simulink model "exampleStorage_type4"  (R2016b)
settings: Solver=ode45  StartTime=0.0  StopTime=3*3600-2  RelTol=1e-3  EnableMultiTasking=on
libraries: carnot x14, simulink x4
settings Model: Creator=drhf  LastModifiedBy=drhf
settings DataIOCC: LimitDataPoints=on  SaveFormat=Array
settings OptimizationCC: ExpressionDepthLimit=2147483647  LifeSpan=inf
settings DebuggingCC: UnderspecifiedInitializationDetection=Classic  MergeDetectMultiDrivingBlocksExec=none  SolverPrmCheckMsg=warning  StateNameClashWarn=warning  SFUnexpectedBacktrackingDiag=warning  SFNoUnconditionalDefaultTransitionDiag=warning  SFExecutionAtInitializationDiag=none
settings HardwareCC: ProdBitPerPointer=32  ProdBitPerSizeT=32  ProdBitPerPtrDiffT=32  ProdLargestAtomicFloat=None  ProdIntDivRoundTo=Undefined  ProdEndianess=Unspecified  ProdWordSize=32  ProdHWDeviceType=32-bit Generic
settings ModelReferenceCC: PropagateSignalLabelsOutOfModel=off
settings GRTTargetCC: TargetLangStandard=C89/C90 (ANSI)  GeneratePreprocessorConditionals=Disable all  CombineOutputUpdateFcns=off  GRTInterface=on
settings ConfigComp: CovMetricSettings=dw  CovHtmlReporting=on  CovSaveCumulativeToWorkspaceVar=on  CovSaveSingleToWorkspaceVar=on  CovExternalEMLEnable=off

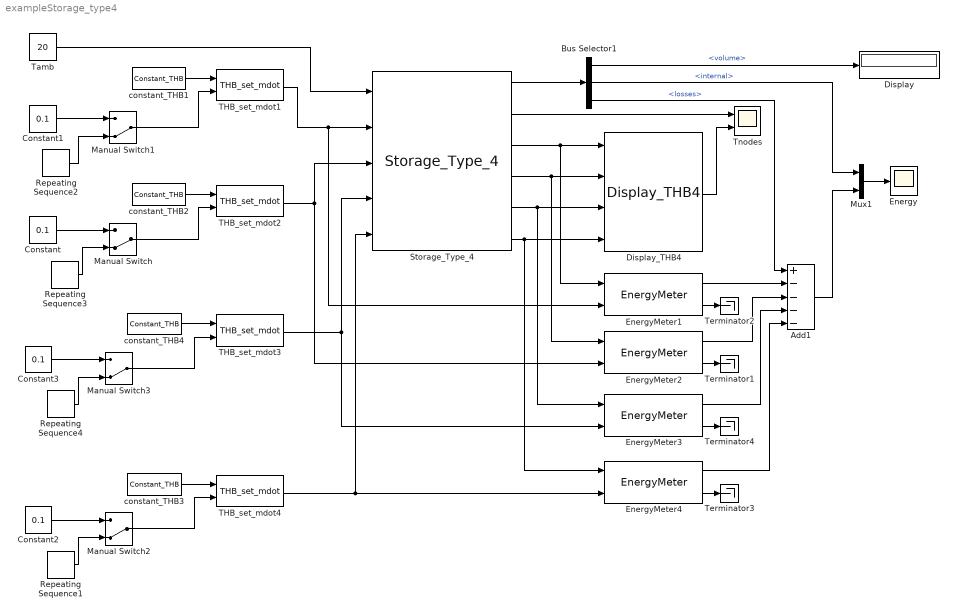
== system exampleStorage_type4 ==
  Add1 : Sum  Inputs=+----
  Bus Selector1 : BusSelector  OutputSignals=volume,energy.internal,energy.losses
  Constant{,1..3} (4 alike) : Constant  Value=0.1
  Display : Display
  Display_THB4 : carnot/Outputs/Display_THB4  t=off  m=on  p=off  id=off  mix=off  d=off
  Energy : Scope
  EnergyMeter{1..4} (4 alike) : carnot/Control/EnergyMeter
  Manual Switch{,1..3} (4 alike) : ManualSwitch  CurrentSetting=0
  Mux1 : Mux  Inputs=2
  Repeating Sequence1 : simulink/Sources/Repeating Sequence  rep_seq_t=[ 0 3600 3600+eps(3600) 7200 7200+eps(7200) 10800]  rep_seq_y=[ 0.12 0.12 0.11+0*eps(3600) 0.11 0.05+0*eps(7200) 0.05]
  Repeating Sequence2 : simulink/Sources/Repeating Sequence  rep_seq_t=[ 0 3600 3600+eps(3600) 7200 7200+eps(7200) 10440 10440+eps(10440) 11160]  rep_seq_y=[ 0 0 0.05+0*eps(3600) 0.05 0.2+0*eps(7200) 0.2 0+0*eps(10440) 0]
  Repeating Sequence3 : simulink/Sources/Repeating Sequence  rep_seq_t=[ 0 3600 3600+eps(3600) 7200 7200+eps(7200) 10800]  rep_seq_y=[ 0 0 0.1+0*eps(3600) 0.1 0.15+0*eps(7200) 0.15]
  Repeating Sequence4 : simulink/Sources/Repeating Sequence  rep_seq_t=[ 0 3600 3600+eps(3600) 7200 7200+eps(7200) 10800]  rep_seq_y=[ 0.11 0.11 0.1+0*eps(3600) 0.1 0.11+0*eps(7200) 0.11]
  Storage_Type_4 : carnot/Storage/Thermal/Storage_Type_4  uloss=0.74  ubot=1.37  utop=0.74  cond=0.62  volume=0.75  dia=0.79  pos=standing cylinder  h_in1=1  h_out1=0.54  dplin1=10  dpqua1=10  h_in2=0.45  h_out2=0  ua0_2=678.6  uam_2=0.411  uat_2=0.287  dplin_2=100  dpqua_2=100  h_in3=0.45  h_out3=0.54  dplin3=10  dpqua3=10  h_in4=0.02  h_out4=0.95  ua0_4=642.2  uam_4=0.369  uat_4=0.684  dplin4=100  dpqua=100  t0=[10:5:55]  nodes=50  mpoints=50
  THB_set_mdot{1..4} (4 alike) : carnot/Source/Simple/THB_set_mdot
  Tamb : Constant  Value=20
  Terminator{1..4} (4 alike) : Terminator
  Tnodes : Scope  NumInputPorts=2
  constant_THB1 : carnot/Source/Simple/Constant_THB  t=15  mdot=0*100/3600  p=1e5  mID=Full Pressure Drop with Static Height  fluid=Water  mix=0  mix2=0  mix3=0  dia=0.02  hgt=0
  constant_THB2 : carnot/Source/Simple/Constant_THB  t=60  mdot=100/3600  p=1e5  mID=Full Pressure Drop with Static Height  fluid=Water  mix=0  mix2=0  mix3=0  dia=0.02  hgt=0
  constant_THB3 : carnot/Source/Simple/Constant_THB  t=40  mdot=100/3600  p=1e5  mID=Full Pressure Drop with Static Height  fluid=Water  mix=0  mix2=0  mix3=0  dia=0.02  hgt=0
  constant_THB4 : carnot/Source/Simple/Constant_THB  t=30  mdot=100/3600  p=1e5  mID=Full Pressure Drop with Static Height  fluid=Water  mix=0  mix2=0  mix3=0  dia=0.02  hgt=0
  wires:
  Bus Selector1/2 -> Mux1/1  "<internal>"
  Tamb/1 -> Storage_Type_4/1
  THB_set_mdot1/1 -> Storage_Type_4/2, EnergyMeter1/2
  THB_set_mdot2/1 -> Storage_Type_4/3, EnergyMeter2/2
  Storage_Type_4/1 -> Bus Selector1/1
  Storage_Type_4/3 -> EnergyMeter1/1, Display_THB4/1
  Storage_Type_4/4 -> EnergyMeter2/1, Display_THB4/2
  Display_THB4/1 -> Tnodes/2
  Mux1/1 -> Energy/1
  EnergyMeter2/2 -> Terminator1/1
  constant_THB1/1 -> THB_set_mdot1/1
  constant_THB2/1 -> THB_set_mdot2/1
  Manual Switch1/1 -> THB_set_mdot1/2
  Manual Switch/1 -> THB_set_mdot2/2
  Constant/1 -> Manual Switch/1
  Repeating Sequence3/1 -> Manual Switch/2
  Constant1/1 -> Manual Switch1/1
  Repeating Sequence2/1 -> Manual Switch1/2
  EnergyMeter1/2 -> Terminator2/1
  Add1/1 -> Mux1/2
  EnergyMeter2/1 -> Add1/3
  EnergyMeter1/1 -> Add1/2
  constant_THB3/1 -> THB_set_mdot4/1
  Manual Switch2/1 -> THB_set_mdot4/2
  Constant2/1 -> Manual Switch2/1
  Repeating Sequence1/1 -> Manual Switch2/2
  THB_set_mdot4/1 -> Storage_Type_4/5, EnergyMeter4/2
  Storage_Type_4/2 -> Tnodes/1
  EnergyMeter4/2 -> Terminator3/1
  Storage_Type_4/6 -> EnergyMeter4/1, Display_THB4/4
  Storage_Type_4/5 -> EnergyMeter3/1, Display_THB4/3
  constant_THB4/1 -> THB_set_mdot3/1
  Manual Switch3/1 -> THB_set_mdot3/2
  Constant3/1 -> Manual Switch3/1
  Repeating Sequence4/1 -> Manual Switch3/2
  THB_set_mdot3/1 -> Storage_Type_4/4, EnergyMeter3/2
  EnergyMeter3/2 -> Terminator4/1
  EnergyMeter3/1 -> Add1/4
  EnergyMeter4/1 -> Add1/5
  Bus Selector1/3 -> Add1/1  "<losses>"
  Bus Selector1/1 -> Display/1  "<volume>"
